simulink model "solvefjalfja"  (R2019a)
settings: Solver=FixedStepAuto  StartTime=0.0  StopTime=0.1  FixedStep=1e-4  RelTol=1e-3
libraries: simulink x3, dspfdesign x2
settings Model: Creator=Sherlock Holmes  LastModifiedBy=Sherlock Holmes

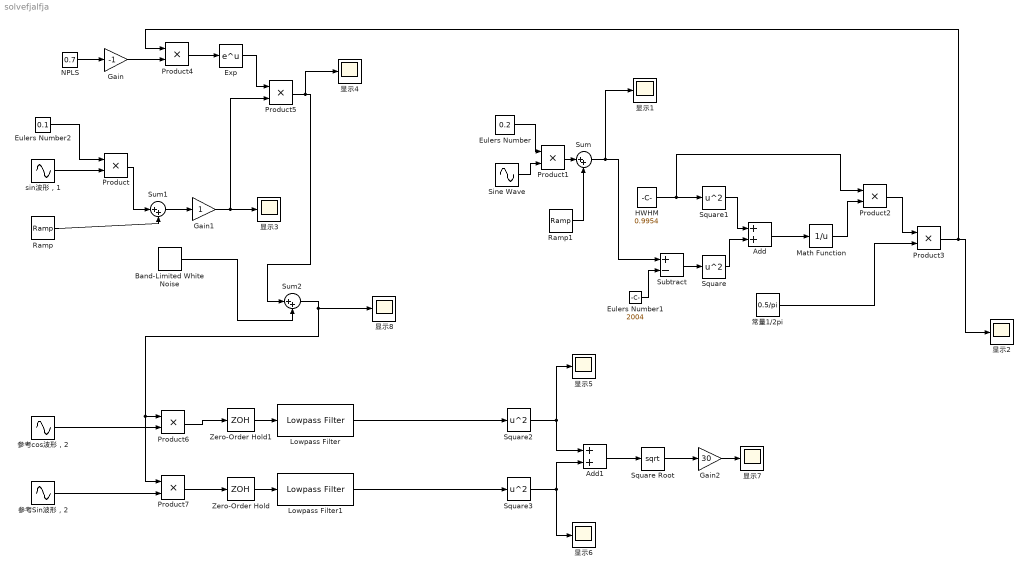
== system solvefjalfja ==
  Add : Sum
  Add1 : Sum
  Band-Limited White Noise : simulink/Sources/Band-Limited White Noise  Cov=[0.1]  Ts=0.1  seed=[23341]
  Eulers Number : Constant  Value=0.2  OutDataTypeStr=Inherit: Inherit via back propagation
  Eulers Number1 : Constant  Value=2004  OutDataTypeStr=Inherit: Inherit via back propagation
  Eulers Number2 : Constant  Value=0.1  OutDataTypeStr=Inherit: Inherit via back propagation
  Exp : Math  SaturateOnIntegerOverflow=on
  Gain : Gain  Gain=-1
  Gain1 : Gain
  Gain2 : Gain  Gain=30
  HWHM : Constant  Value=0.9954  OutDataTypeStr=Inherit: Inherit via back propagation
  Lowpass Filter : dspfdesign/Lowpass Filter  FilterType=FIR  DesignForMinimumOrder=on  FilterOrder=50  PassbandFrequency=1000  StopbandFrequency=1600  PassbandRipple=0.1  StopbandAttenuation=80  InheritSampleRate=off  SampleRate=44100  SimulateUsing=Interpreted execution  roundingMode=Floor  coeffsDataTypeStr=fixdt(1,16)
  Lowpass Filter1 : dspfdesign/Lowpass Filter  FilterType=FIR  DesignForMinimumOrder=on  FilterOrder=50  PassbandFrequency=1000  StopbandFrequency=1600  PassbandRipple=0.1  StopbandAttenuation=80  InheritSampleRate=off  SampleRate=44100  SimulateUsing=Interpreted execution  roundingMode=Floor  coeffsDataTypeStr=fixdt(1,16)
  Math Function : Math  Operator=reciprocal  RndMeth=Zero  SaturateOnIntegerOverflow=on
  NPLS : Constant  Value=0.7  OutDataTypeStr=Inherit: Inherit via back propagation
  Product{,1..7} (8 alike) : Product
  Ramp : simulink/Sources/Ramp  slope=20  start=0  InitialOutput=2
  Ramp1 : simulink/Sources/Ramp  slope=80  start=0  InitialOutput=2000
  Sine Wave : Sin  Frequency=5000  SampleTime=0
  Square{,1..3} (4 alike) : Math  Operator=square  SaturateOnIntegerOverflow=on
  Square Root : Sqrt  SaturateOnIntegerOverflow=on
  Subtract : Sum  Inputs=+-
  Sum : Sum  Inputs=|++
  Sum1 : Sum  Inputs=|++
  Sum2 : Sum  Inputs=|++
  Zero-Order Hold : ZeroOrderHold  SampleTime=-1
  Zero-Order Hold1 : ZeroOrderHold  SampleTime=-1
  sin波形，1 : Sin  Frequency=5000  SampleTime=0
  参考Sin波形，2 : Sin  Frequency=10000  SampleTime=0
  参考cos波形，2 : Sin  Frequency=10000  Phase=90  SampleTime=0
  常量1/2pi : Constant  Value=0.5/pi  OutDataTypeStr=Inherit: Inherit via back propagation
  显示{1..8} (8 alike) : Scope
  wires:
  sin波形，1/1 -> Product/2
  Eulers Number/1 -> Product1/1
  Sine Wave/1 -> Product1/2
  Product1/1 -> Sum/1
  Sum/1 -> 显示1/1, Subtract/1
  Eulers Number1/1 -> Subtract/2
  Subtract/1 -> Square/1
  HWHM/1 -> Product2/1, Square1/1
  Square1/1 -> Add/1
  Square/1 -> Add/2
  Add/1 -> Math Function/1
  Math Function/1 -> Product2/2
  Product2/1 -> Product3/1
  常量1/2pi/1 -> Product3/2
  Product3/1 -> Product4/1, 显示2/1
  Eulers Number2/1 -> Product/1
  Product/1 -> Sum1/1
  Ramp/1 -> Sum1/2
  Sum1/1 -> Gain1/1
  NPLS/1 -> Gain/1
  Gain/1 -> Product4/2
  Gain1/1 -> Product5/2, 显示3/1
  Product4/1 -> Exp/1
  Exp/1 -> Product5/1
  Product5/1 -> 显示4/1, Sum2/1
  Band-Limited White Noise/1 -> Sum2/2
  参考cos波形，2/1 -> Product6/2
  参考Sin波形，2/1 -> Product7/2
  Sum2/1 -> Product6/1, Product7/1, 显示8/1
  Product6/1 -> Zero-Order Hold1/1
  Product7/1 -> Zero-Order Hold/1
  Zero-Order Hold1/1 -> Lowpass Filter/1
  Zero-Order Hold/1 -> Lowpass Filter1/1
  Lowpass Filter1/1 -> Square3/1
  Lowpass Filter/1 -> Square2/1
  Square2/1 -> 显示5/1, Add1/1
  Square3/1 -> 显示6/1, Add1/2
  Add1/1 -> Square Root/1
  Ramp1/1 -> Sum/2
  Gain2/1 -> 显示7/1
  Square Root/1 -> Gain2/1
